simulink model "ESTS_TFY_FLatTir_test"  (R2023b)
settings: Solver=VariableStepAuto  StartTime=0.0  StopTime=10.0  RelTol=1e-3
libraries: ESTS_TFY_FLatTir x1
settings Model: Creator=blatak  LastModifiedBy=blatak

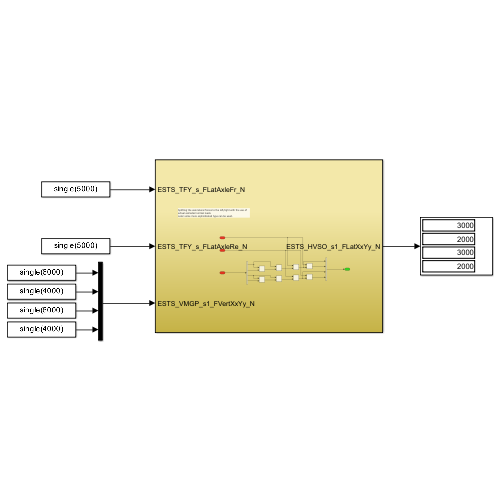
[thumbnail: Simulink's stored preview of the top-level diagram]
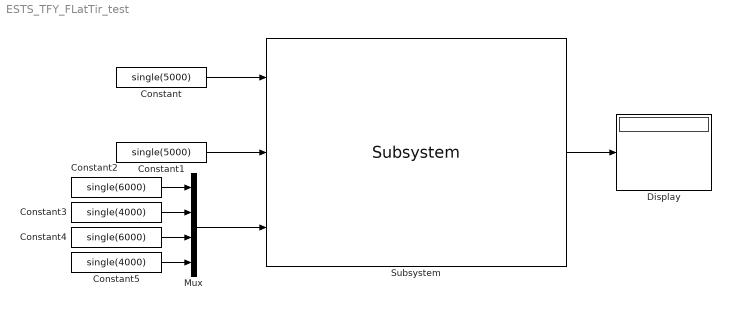
== system ESTS_TFY_FLatTir_test ==
  Constant : Constant  Value=single(5000)
  Constant1 : Constant  Value=single(5000)
  Constant2 : Constant  Value=single(6000)
  Constant3 : Constant  Value=single(4000)
  Constant4 : Constant  Value=single(6000)
  Constant5 : Constant  Value=single(4000)
  Display : Display
  Mux : Mux
  Subsystem : ESTS_TFY_FLatTir/Subsystem  SystemSampleTime=-1  VariantActivationTime=update diagram  AllowFlexibleInterface=on  Latency=0  AutoFrameSizeCalculation=off
  wires:
  Constant1/1 -> Subsystem/2
  Constant/1 -> Subsystem/1
  Constant5/1 -> Mux/4
  Constant3/1 -> Mux/2
  Constant2/1 -> Mux/1
  Mux/1 -> Subsystem/3
  Constant4/1 -> Mux/3
  Subsystem/1 -> Display/1
